simulink model "system_sim_test2"  (R2015a)
settings: Solver=ode45  StartTime=0.0  StopTime=3600  FixedStep=0.05  RelTol=1e-3
values from neighbouring files (symbols this model uses):
  area = 1.2    [run_sim_auto.m]    (also in run_sim_test4.m = 2; sim_testing.m; wrkspc_no_1.mat; wrkspc_no_10.mat)
  Cd = 0.6    [run_sim_auto.m]    (also in run_sim_test4.m = 1; sim_testing.m; wrkspc_no_1.mat; wrkspc_no_10.mat)
  Crr = 0.005    [run_sim_test4.m]    (also in wrkspc_no_1.mat; wrkspc_no_10.mat; wrkspc_no_18.mat; wrkspc_no_22.mat)
  g = 9.81    [run_sim.m]    (also in run_sim_auto.m; run_sim_test.m; run_sim_test4.m; run_sim_v2.m)
  m = 210    [run_sim_auto.m]    (also in run_sim_test4.m = 150; sim_testing.m; wrkspc_no_1.mat; wrkspc_no_10.mat)
  rho_air = 1.225    [run_sim.m]    (also in run_sim_auto.m; run_sim_test.m; run_sim_test4.m; run_sim_v2.m)
settings Model: Creator=marco  LastModifiedBy=marco

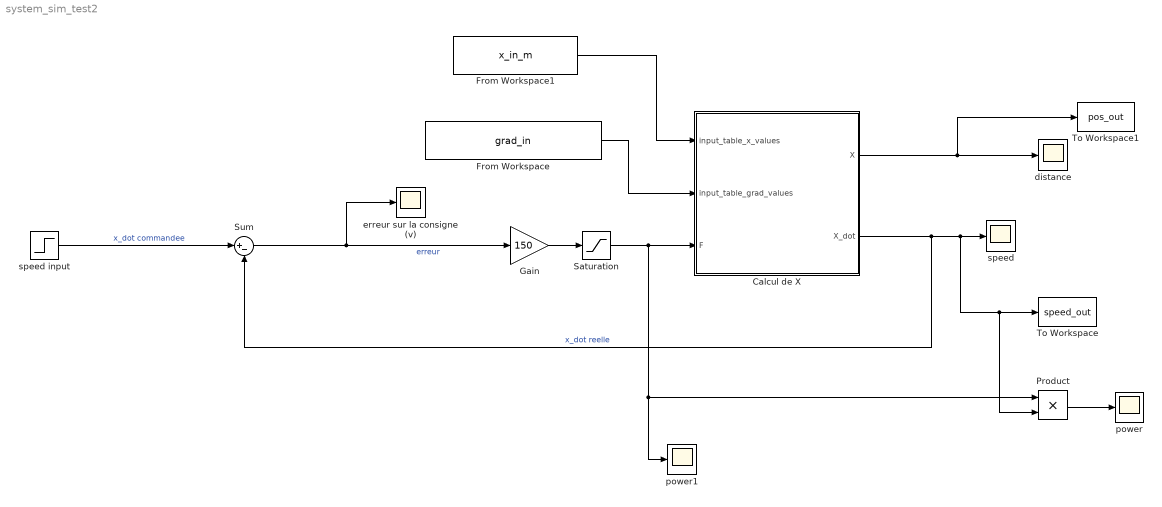
== system system_sim_test2 ==
  Calcul de X : Subsystem
  From Workspace : FromWorkspace  VariableName=grad_in  SampleTime=0
  From Workspace1 : FromWorkspace  VariableName=x_in_m  SampleTime=0
  Gain : Gain  Gain=150
  Product : Product
  Saturation : Saturate  UpperLimit=200  LowerLimit=-200
  Sum : Sum  Inputs=|+-
  To Workspace : ToWorkspace  VariableName=speed_out  SampleTime=-1
      settings: Save2DSignal=2-D array (concatenate along first dimension)
  To Workspace1 : ToWorkspace  VariableName=pos_out  SampleTime=-1
      settings: Save2DSignal=2-D array (concatenate along first dimension)
  distance : Scope
  erreur sur la consigne (v) : Scope
      settings: SaveName=ScopeData6
  power : Scope
      settings: SaveName=ScopeData4
  power1 : Scope
      settings: TimeRange=60  YMin=4  YMax=5.5  SaveName=ScopeData5
  speed : Scope
  speed input : Step  Time=0.1  After=4.16  SampleTime=1
  wires:
  Calcul de X/2(X_dot) -> Sum/2, Product/2, To Workspace/1, speed/1  "x_dot reelle"
  Calcul de X/1(X) -> To Workspace1/1, distance/1
  speed input/1 -> Sum/1  "x_dot commandee"
  From Workspace1/1 -> Calcul de X/1(input_table_x_values)
  From Workspace/1 -> Calcul de X/2(input_table_grad_values)
  Product/1 -> power/1
  Saturation/1 -> Product/1, power1/1, Calcul de X/3(F)
  Sum/1 -> erreur sur la consigne (v)/1, Gain/1  "erreur"
  Gain/1 -> Saturation/1

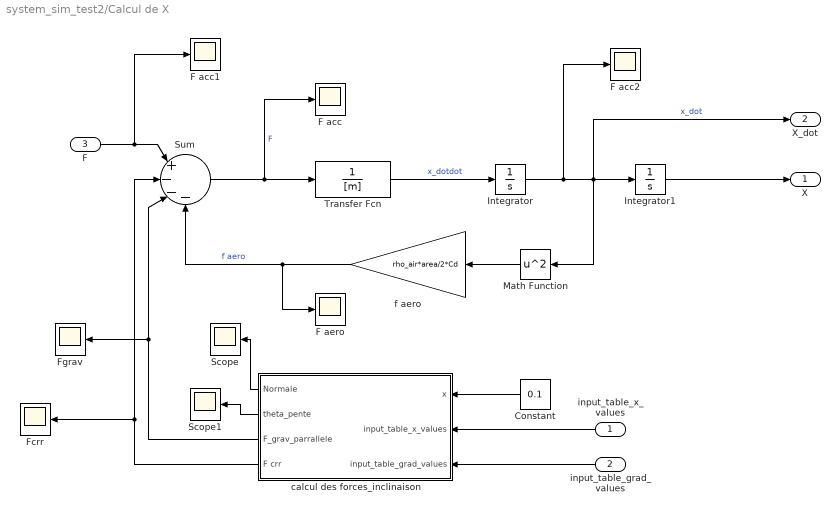
== system system_sim_test2/Calcul de X ==
  input_table_x_values : Inport
  input_table_grad_values : Inport  Port=2
  F : Inport  Port=3
  Constant : Constant  Value=0.1
  F acc : Scope
      settings: SaveName=ScopeData7
  F acc1 : Scope
      settings: SaveName=ScopeData12
  F acc2 : Scope
      settings: SaveName=ScopeData13
  F aero : Scope
      settings: SaveName=ScopeData14
  Fcrr : Scope
      settings: SaveName=ScopeData10
  Fgrav : Scope
      settings: SaveName=ScopeData9
  Integrator : Integrator
  Integrator1 : Integrator
  Math Function : Math  Operator=square  SaturateOnIntegerOverflow=on
  Scope : Scope
      settings: SaveName=ScopeData2
  Scope1 : Scope
      settings: SaveName=ScopeData3
  Sum : Sum  Inputs=|+---
  Transfer Fcn : TransferFcn  Denominator=[m]
  calcul des forces_inclinaison : Subsystem
  f aero : Gain  Gain=rho_air*area/2*Cd
  X : Outport
  X_dot : Outport  Port=2
  wires:
  Sum/1 -> F acc/1, Transfer Fcn/1  "F"
  Transfer Fcn/1 -> Integrator/1  "x_dotdot"
  Integrator/1 -> F acc2/1, Math Function/1, X_dot/1, Integrator1/1  "x_dot"
  f aero/1 -> F aero/1, Sum/4  "f aero"
  F/1 -> F acc1/1, Sum/1
  calcul des forces_inclinaison/3(F_grav_parrallele) -> Fgrav/1, Sum/3
  calcul des forces_inclinaison/4(F crr) -> Fcrr/1, Sum/2
  input_table_x_values/1 -> calcul des forces_inclinaison/2(input_table_x_values)
  input_table_grad_values/1 -> calcul des forces_inclinaison/3(input_table_grad_values)
  Integrator1/1 -> X/1
  calcul des forces_inclinaison/1(Normale) -> Scope/1
  calcul des forces_inclinaison/2(theta_pente) -> Scope1/1
  Math Function/1 -> f aero/1
  Constant/1 -> calcul des forces_inclinaison/1(x)

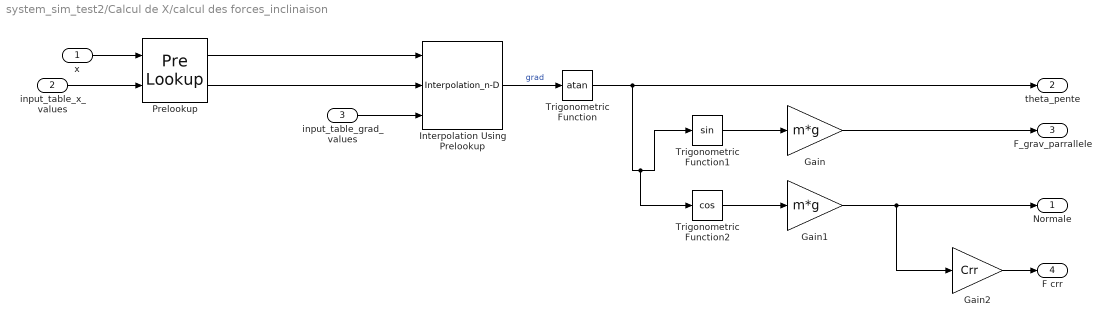
== system system_sim_test2/Calcul de X/calcul des forces_inclinaison ==
  x : Inport
  input_table_x_values : Inport  Port=2
  input_table_grad_values : Inport  Port=3
  Gain : Gain  Gain=m*g
  Gain1 : Gain  Gain=m*g
  Gain2 : Gain  Gain=Crr
  Interpolation Using Prelookup : Interpolation_n-D  NumberOfTableDimensions=1  TableSource=Input port  InternalRulePriority=Speed
      settings: InputPortMap=u0,u1,p2
  Prelookup : PreLookup  BreakpointsDataSource=Input port  BreakpointsData=[10:10:110]  ExtrapMethod=Linear
      settings: InputPortMap=u0,p1
  Trigonometric Function : Trigonometry  Operator=atan
  Trigonometric Function1 : Trigonometry
  Trigonometric Function2 : Trigonometry  Operator=cos
  Normale : Outport
  theta_pente : Outport  Port=2
  F_grav_parrallele : Outport  Port=3
  F crr : Outport  Port=4
  wires:
  x/1 -> Prelookup/1
  Interpolation Using Prelookup/1 -> Trigonometric Function/1  "grad"
  Trigonometric Function1/1 -> Gain/1
  Trigonometric Function2/1 -> Gain1/1
  Gain1/1 -> Gain2/1, Normale/1
  Gain/1 -> F_grav_parrallele/1
  Gain2/1 -> F crr/1
  Prelookup/1 -> Interpolation Using Prelookup/1
  Prelookup/2 -> Interpolation Using Prelookup/2
  input_table_grad_values/1 -> Interpolation Using Prelookup/3
  input_table_x_values/1 -> Prelookup/2
  Trigonometric Function/1 -> Trigonometric Function2/1, Trigonometric Function1/1, theta_pente/1
